simulink model "doubleint"  (R2015b)
settings: Solver=ode4  StartTime=0.0  StopTime=2.1  FixedStep=10^-4  MaxStep=0.2  RelTol=1e-3
settings Model: Creator=Gautham  LastModifiedBy=Gautham

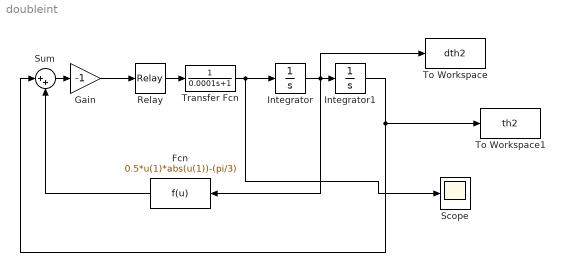
== system doubleint ==
  Fcn : Fcn  Expr=0.5*u(1)*abs(u(1))-(pi/3)
  Gain : Gain  Gain=-1
  Integrator : Integrator
  Integrator1 : Integrator
  Relay : Relay  OffOutputValue=-1
  Scope : Scope
  Sum : Sum  Inputs=|++
  To Workspace : ToWorkspace  VariableName=dth2  SampleTime=-1
  To Workspace1 : ToWorkspace  VariableName=th2  SampleTime=-1
  Transfer Fcn : TransferFcn  Denominator=[0.0001 1]
  wires:
  Integrator/1 -> To Workspace/1, Fcn/1, Integrator1/1
  Gain/1 -> Relay/1
  Sum/1 -> Gain/1
  Integrator1/1 -> To Workspace1/1, Sum/1
  Fcn/1 -> Sum/2
  Relay/1 -> Transfer Fcn/1
  Transfer Fcn/1 -> Integrator/1, Scope/1
